simulink model "high_level_magnetorquer_controller"  (R2025b)
settings: Solver=VariableStepAuto  StartTime=0.0  StopTime=10.0  RelTol=1e-3
settings Model: Creator=taizo  LastModifiedBy=taizo

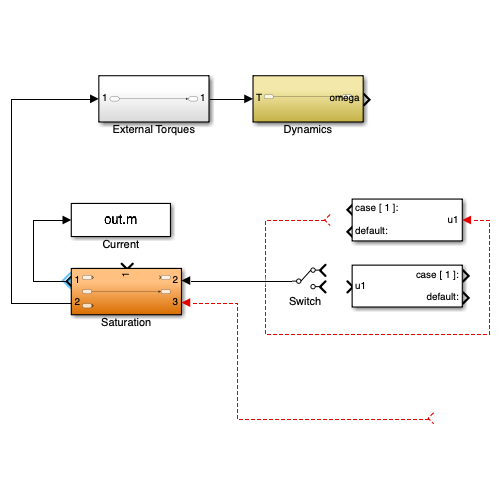
[thumbnail: Simulink's stored preview of the top-level diagram]
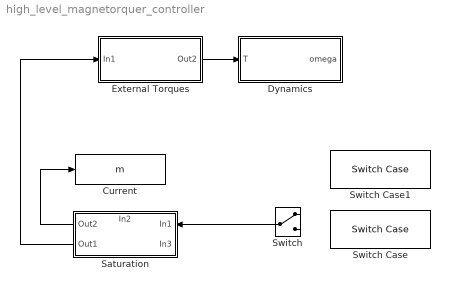
== system high_level_magnetorquer_controller ==
  Current : ToWorkspace  VariableName=m  SaveFormat=Timeseries  SampleTime=-1
  Dynamics : Subsystem
  External Torques : Subsystem
  Saturation : Subsystem
      settings: PortSchema="{\"entries\":[{\"content\":{\"sides\":[{\"content\":{\"connectorIds\":[\"Out1\",\"Out2\"]},\"type\":\"ConnectorPlacement.EquallySpacedRectSide\",\"uuid\":\"d640583f-223f-4ad6-b0d1-6fc6ddb27c15\"},{\"content\":{\"connectorIds\":[\"In2\",\"In3\"],\"side\":\"RIGHT\"},\"type\":\"ConnectorPlacement.EquallySpacedRectSide\",\"uuid\":\"3044df4b-5357-4895-84a3-f300a7f5b3c9\"},{\"content\":{\"connectorIds\":[\"In1\"],\"side\":\"TOP\"},\"type\":\"ConnectorPlacement.EquallySpacedRectSide\",\"uuid\":\"f19897f3-1a11-4567-824e-82b12d082443\"},{\"content\":{\"side\":\"BOTTOM\"},\"type\":\"ConnectorPlacement.EquallySpacedRectSide\",\"uuid\":\"9e1d27e2-c60d-4f92-a216-b062911b593b\"}]},\"type\":\"ConnectorPlacement.EquallySpacedConnector\",\"uuid\":\"5fac82cd-05a3-42d1-a81f-62937d062f68\"}],\"packageUris\":[\"http://schema.mathworks.com/mf0/Connector/R2020b\"],\"version\":\"1.0\"}"
  Switch : ManualSwitch
  Switch Case : SwitchCase
  Switch Case1 : SwitchCase
  wires:
  External Torques/1(Out2) -> Dynamics/1(T)
  Saturation/2(Out1) -> External Torques/1(In1)
  Saturation/1(Out2) -> Current/1
  Switch/1 -> Saturation/2(In1)
  ? -> Saturation/3(In3)
  ? -> Switch Case1/1

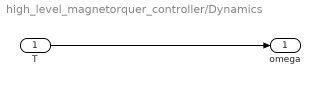
== system high_level_magnetorquer_controller/Dynamics ==
  T : Inport
  omega : Outport
  wires:
  T/1 -> omega/1

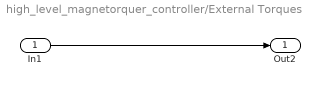
== system high_level_magnetorquer_controller/External Torques ==
  In1 : Inport
  Out2 : Outport
  wires:
  In1/1 -> Out2/1

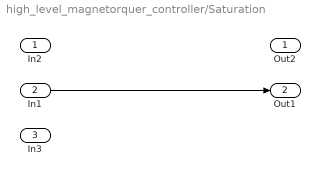
== system high_level_magnetorquer_controller/Saturation ==
  In2 : Inport
  In1 : Inport  Port=2
  In3 : Inport  Port=3
  Out2 : Outport
  Out1 : Outport  Port=2
  wires:
  In1/1 -> Out1/1
